simulink model "FMmod"  (R2023b)
settings: Solver=VariableStepAuto  StartTime=0.0  StopTime=10.0  RelTol=1e-3
libraries: dspsigops x1, simulink x1
settings Model: Creator=garaya  LastModifiedBy=garaya

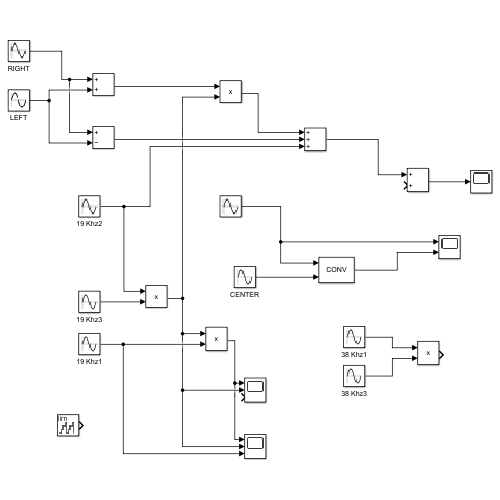
[thumbnail: Simulink's stored preview of the top-level diagram]
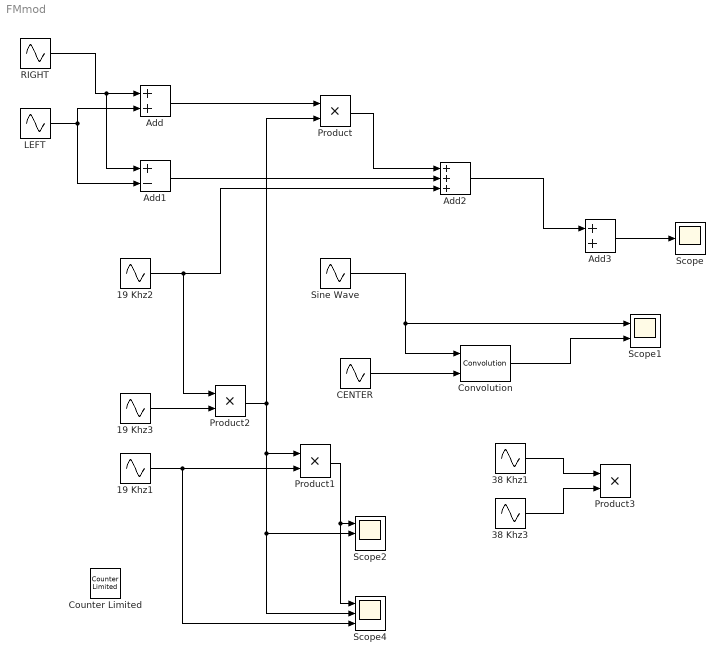
== system FMmod ==
  19 Khz1 : Sin  Frequency=33  SampleTime=0
  19 Khz2 : Sin  Frequency=33  SampleTime=0
  19 Khz3 : Sin  Frequency=33  SampleTime=0
  38 Khz1 : Sin  Frequency=66  SampleTime=0
  38 Khz3 : Sin  Frequency=66  Phase=1.5708  SampleTime=0
  Add : Sum
  Add1 : Sum  Inputs=+-
  Add2 : Sum  Inputs=+++
  Add3 : Sum
  CENTER : Sin  Frequency=200  SampleTime=0
  Convolution : dspsigops/Convolution  domain=Frequency  roundingMode=Floor  overflowMode=off  outputDataTypeStr=Inherit: Same as accumulator  outputMin=[]  outputMax=[]  outputLastDataTypeStr=Inherit: Same as accumulator
  Counter Limited : simulink/Sources/Counter Limited  uplimit=7  tsamp=-1
  LEFT : Sin  Frequency=200  SampleTime=0
  Product{,1..3} (4 alike) : Product
  RIGHT : Sin  Frequency=100  SampleTime=0
  Scope : Scope
  Scope1 : Scope  NumInputPorts=2
  Scope2 : Scope  NumInputPorts=3
  Scope4 : Scope  NumInputPorts=3
  Sine Wave : Sin  Frequency=99  SampleTime=0
  wires:
  LEFT/1 -> Add/2, Add1/2
  RIGHT/1 -> Add1/1, Add/1
  Add1/1 -> Add2/2
  Add/1 -> Product/1
  Product/1 -> Add2/1
  19 Khz2/1 -> Product2/1, Add2/3
  CENTER/1 -> Convolution/2
  Add2/1 -> Add3/1
  Add3/1 -> Scope/1
  Sine Wave/1 -> Scope1/1, Convolution/1
  Convolution/1 -> Scope1/2
  Product2/1 -> Scope4/2, Scope2/2, Product1/1, Product/2
  Product1/1 -> Scope4/1, Scope2/1
  38 Khz1/1 -> Product3/1
  38 Khz3/1 -> Product3/2
  19 Khz3/1 -> Product2/2
  19 Khz1/1 -> Scope4/3, Product1/2
